simulink model "Pacemaker_Main_Stateflow"  (R2020a)
settings: Solver=FixedStepAuto  StartTime=0.0  StopTime=10.0  FixedStep=1e-3  RelTol=1e-3  EnableMultiTasking=on
undefined symbols (not defined in the file): D0, D10, D11, D2, D5, D8, PTA0, PTA2, PTB9, PTC16, PTD0, PTD2
libraries: frdmk64flib x9
settings Model: ExtModeTrigDuration=5  Creator=forre  LastModifiedBy=Kevin
settings OptimizationCC: EnhancedBackFolding=on  PassReuseOutputArgsAs=Individual arguments  ZeroExternalMemoryAtStartup=off  ZeroInternalMemoryAtStartup=off  MaxStackSize=64  OptimizeBlockOrder=speed  DifferentSizesBufferReuse=on  OptimizationCustomize=off  EfficientTunableParamExpr=on
settings DebuggingCC: ParameterTunabilityLossMsg=error
settings HardwareCC: ProdBitPerPointer=32  ProdBitPerSizeT=32  ProdBitPerPtrDiffT=32  ProdLargestAtomicInteger=Long  ProdLargestAtomicFloat=Double  ProdWordSize=32  ProdHWDeviceType=ARM Compatible->ARM Cortex
settings SFSimCC: MATLABDynamicMemAlloc=off
settings RTWCC: SystemTargetFile=ert.tlc  HardwareBoard=NXP FRDM-K64F  TemplateMakefile=ert_default_tmf  Toolchain=GNU Tools for ARM Embedded Processors
settings CodeAppCC: ForceParamTrailComments=on  IgnoreCustomStorageClasses=off  OperatorAnnotations=on  SimulinkDataObjDesc=on  SFDataObjDesc=on  InsertBlockDesc=on

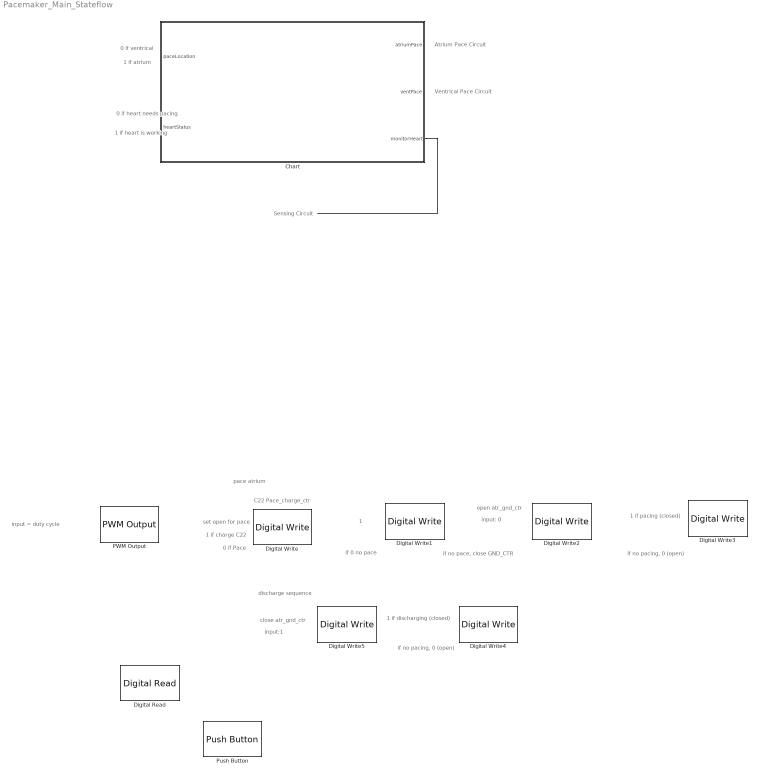
== system Pacemaker_Main_Stateflow ==
  note: Sensing Circuit
  note: Atrium Pace Circuit
  note: 0 if heart needs
      | pacing
  note: 0 if ventrical
  note: 1 if atrium
  note: input = duty cycle
  note: set open for pace
  note: discharge sequence
  note: if no pacing, 0 (open)
  note: 1 if pacing (closed)
  note: if no pace, close GND_CTR
  note: input: 0
  note: open atr_gnd_ctr
  note: if 0 no pace
  note: 1
  note: pace atrium
  note: 0 if Pace
  note: 1 if charge C22
  note: C22 Pace_charge_ctr
  note: if no pacing, 0 (open)
  note: 1 if discharging (closed)
  note: input:1
  note: close atr_gnd_ctr
  note: Ventrical Pace Circuit
  note: 1 if heart is
      | working
  Chart : Stateflow chart  TreatAsAtomicUnit=on
  Digital Read : frdmk64flib/Digital Read  Whichpin=PTC16 (D0)  SampleTime=-1
  Digital Write : frdmk64flib/Digital Write  Whichpin=PTB9 (D2)
  Digital Write1 : frdmk64flib/Digital Write  Whichpin=PTA0 (D8)
  Digital Write2 : frdmk64flib/Digital Write  Whichpin=PTD2 (D11)
  Digital Write3 : frdmk64flib/Digital Write  Whichpin=PTD0 (D10)
  Digital Write4 : frdmk64flib/Digital Write  Whichpin=PTD0 (D10)
  Digital Write5 : frdmk64flib/Digital Write  Whichpin=PTD2 (D11)
  PWM Output : frdmk64flib/PWM Output  Whichpin=PTA2 (D5)  InitialFrequency=1000  InitialDutyCycle=50
  Push Button : frdmk64flib/Push Button  Whichswitch=SW2  SampleTime1=-1
  wires:
  ? -> PWM Output/1
  Chart/3(monitorHeart) -> ?
  ? -> Chart/1(paceLocation), Chart/2(heartStatus)

== stateflow chart Pacemaker_Main_Stateflow/Chart ==
  state HEART_MONITORING
    entry:
    monitorHeart = True;
    ventPace = False;
    atriumPace = False;
  state VENTRICAL_PACE
    entry:
    monitorHeart = False;
    atriumPace = False;
    ventPace = True;
  state ATRIUM_PACE
    entry:
    monitorHeart = False;
    atriumPace = True;
    ventPace = False;
  (default) -> HEART_MONITORING
  HEART_MONITORING -> HEART_MONITORING [order 2] : [heartStatus == 1]
  HEART_MONITORING -> ATRIUM_PACE [order 1] : [paceLocation == 1 && heartStatus == 0]
  HEART_MONITORING -> VENTRICAL_PACE [order 3] : [paceLocation == 0 && heartStatus == 0]
  VENTRICAL_PACE -> HEART_MONITORING : after(10,sec)
  ATRIUM_PACE -> HEART_MONITORING : after(10,sec)
  data: paceLocation input int8; atriumPace output boolean; ventPace output boolean; monitorHeart output int8; heartStatus input int8
